simulink model "HouseHolderTransformTest"  (R2023b)
settings: Solver=VariableStepAuto  StartTime=0.0  StopTime=1  FixedStep=0.0038461538461538464  RelTol=1e-3
values from neighbouring files (symbols this model uses):
  A = [0.588528123101 -3.46944695195e-18 -8.67361737988e-19 0 0 6.93889390391e-18 6.93889390391e-18 6.93889390391e-18 1.38777878078e-17 0 0 6.93889390391e-18 ... (1040 elements, 260x4)]    [InitData.mat]
undefined symbols (not defined in the file or in its folder): FrameLength, NumOfAntennas
libraries: hdlsllib x5, dspstat3 x5
(part 1 of 2)
settings Model: Creator=Koche  LastModifiedBy=Koche
settings DebuggingCC: UnderSpecifiedDimensionMsg=error

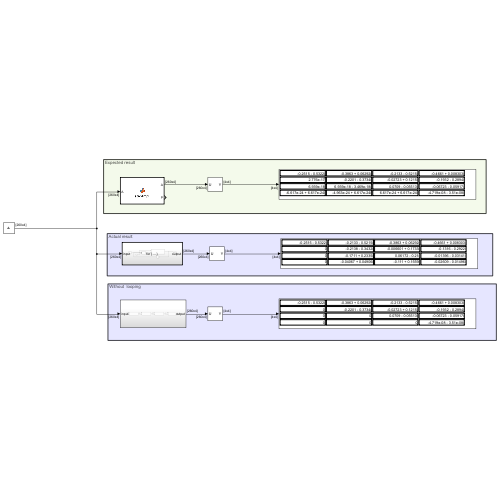
[thumbnail: Simulink's stored preview of the top-level diagram]
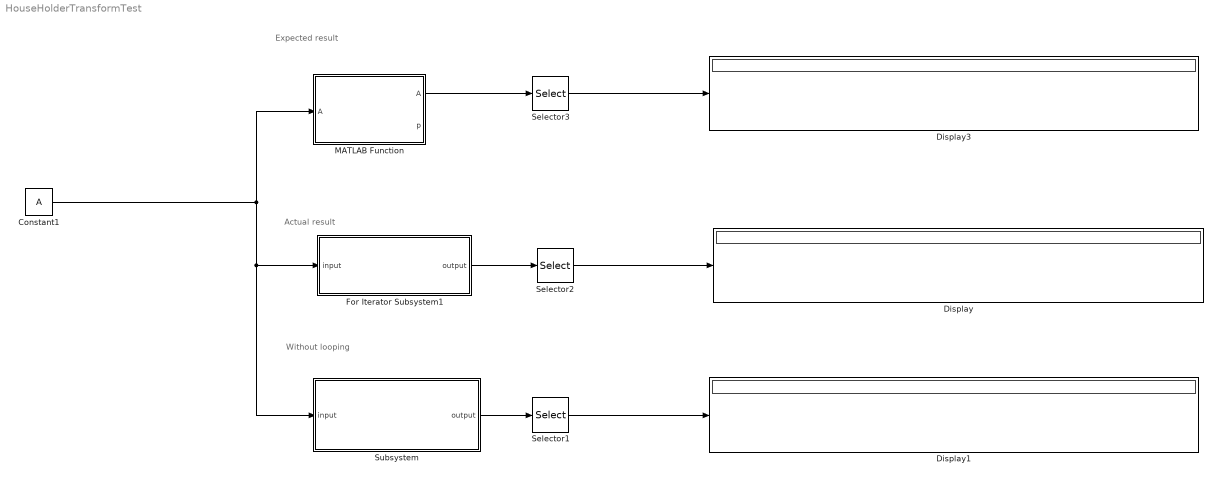
== system HouseHolderTransformTest ==
  note: Without looping
  note: Expected result
  note: Actual result
  Constant1 : Constant  Value=A  SampleTime=1/FrameLength
  Display : Display
  Display1 : Display
  Display3 : Display
  For Iterator Subsystem1 : Subsystem  TreatAsAtomicUnit=on
  MATLAB Function : MATLAB Function  TreatAsAtomicUnit=on
  Selector1 : Selector  NumberOfDimensions=2  InputPortWidth=3  IndexOptions=Index vector (dialog),Index vector (dialog)  Indices=[1 2 3 4],[1 2 3 4]  OutputSizes=1,1
  Selector2 : Selector  NumberOfDimensions=2  InputPortWidth=3  IndexOptions=Index vector (dialog),Index vector (dialog)  Indices=[1 2 3 4],[1 2 3 4]  OutputSizes=1,1
  Selector3 : Selector  NumberOfDimensions=2  InputPortWidth=3  IndexOptions=Index vector (dialog),Index vector (dialog)  Indices=[1 2 3 4],[1 2 3 4]  OutputSizes=1,1
  Subsystem : Subsystem
  wires:
  Constant1/1 -> Subsystem/1(input), For Iterator Subsystem1/1(input), MATLAB Function/1("A ")
  For Iterator Subsystem1/1(output) -> Selector2/1
  Selector2/1 -> Display/1
  Selector3/1 -> Display3/1
  MATLAB Function/1(A) -> Selector3/1
  Subsystem/1(output) -> Selector1/1
  Selector1/1 -> Display1/1

== system HouseHolderTransformTest/For Iterator Subsystem1 ==
  input : Inport
  For Iterator : ForIterator  IterationLimit=NumOfAntennas
  Memory1 : Memory  InheritSampleTime=on
  Subsystem3 : Subsystem
  Switch1 : Switch  Criteria=u2 > Threshold  Threshold=1  SaturateOnIntegerOverflow=off  InputSameDT=off
  output : Outport
  wires:
  input/1 -> Switch1/3
  Memory1/1 -> Switch1/1
  Switch1/1 -> Subsystem3/2(input)
  For Iterator/1 -> Subsystem3/1(n), Switch1/2
  Subsystem3/1(output) -> Memory1/1, output/1

== system HouseHolderTransformTest/Subsystem ==
  input : Inport
  Constant : Constant  OutDataTypeStr=int32
  Constant1 : Constant  Value=2  OutDataTypeStr=int32
  Constant2 : Constant  Value=3  OutDataTypeStr=int32
  Constant3 : Constant  Value=4  OutDataTypeStr=int32
  Subsystem1 : Subsystem
  Subsystem2 : Subsystem
  Subsystem3 : Subsystem
  Subsystem4 : Subsystem
  output : Outport
  wires:
  Constant/1 -> Subsystem3/1(n)
  Subsystem3/1(output) -> Subsystem1/2(input)
  Constant2/1 -> Subsystem2/1(n)
  Subsystem4/1(output) -> output/1
  Subsystem2/1(output) -> Subsystem4/2(input)
  Subsystem1/1(output) -> Subsystem2/2(input)
  input/1 -> Subsystem3/2(input)
  Constant3/1 -> Subsystem4/1(n)
  Constant1/1 -> Subsystem1/1(n)

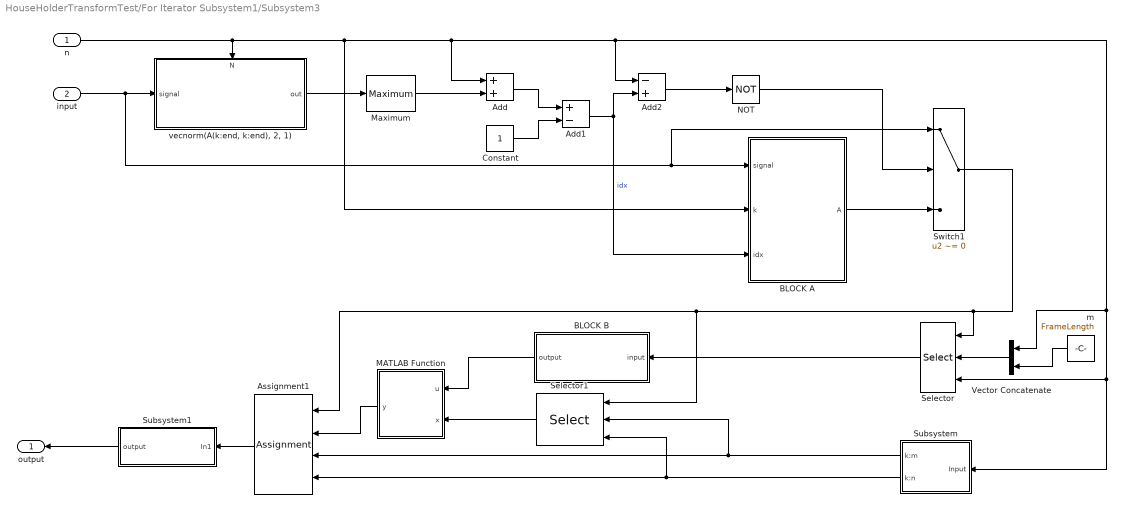
== system HouseHolderTransformTest/For Iterator Subsystem1/Subsystem3 ==
  n : Inport
  input : Inport  Port=2
  Add : Sum
  Add1 : Sum  Inputs=+-
  Add2 : Sum  Inputs=-+
  Assignment1 : Assignment  NumberOfDimensions=2  IndexOptions=Index vector (port),Index vector (port)  Indices=1,1  OutputSizes=1,1
  BLOCK A : Subsystem  TreatAsAtomicUnit=on
  BLOCK B : Subsystem
  Constant : Constant  SampleTime=-1
  MATLAB Function : MATLAB Function  TreatAsAtomicUnit=on
  Maximum : dspstat3/Maximum  operation=maximum  fcn=Index  indexBase=One  operateOver=Each column  Dimension=1  InputProcessing=Columns as channels (frame based)  reset=None  roiEnable=off  roiType=Rectangles  roiPortion=Entire ROI  roiOutput=Individual statistics for each ROI  roiFlag=off  roundingMode=Floor  overflowMode=off  accumDataTypeStr=Inherit: Same as product output  accumLastDataTypeStr=Inherit: Same as product output
      settings: LibrarySourceBlock=dsphdlsupportstat/Maximum
  NOT : Logic  Operator=NOT  IconShape=distinctive  AllPortsSameDT=off  OutDataTypeStr=boolean
  Selector : Selector  NumberOfDimensions=2  InputPortWidth=3  IndexOptions=Starting and ending indices (port),Index vector (port)  Indices=[1 3],1  OutputSizes=1,1
  Selector1 : Selector  NumberOfDimensions=2  InputPortWidth=3  IndexOptions=Index vector (port),Index vector (port)  Indices=[1 3],1  OutputSizes=1,1
  Subsystem : Subsystem
  Subsystem1 : Subsystem
  Switch1 : Switch  Criteria=u2 ~= 0  SaturateOnIntegerOverflow=off  InputSameDT=off
  Vector Concatenate : Concatenate
  m : Constant  Value=FrameLength  OutDataTypeStr=int32
  "vecnorm(A(k:end, k:end), 2, 1)" : Subsystem
      settings: PortSchema="{\"entries\":[{\"content\":{\"sides\":[{\"content\":{\"connectorIds\":[\"In1\"]},\"type\":\"ConnectorPlacement.EquallySpacedRectSide\",\"uuid\":\"ddbbb4e8-2c6c-4e6c-8e2e-3b3671634aad\"},{\"content\":{\"connectorIds\":[\"Out1\"],\"side\":\"RIGHT\"},\"type\":\"ConnectorPlacement.EquallySpacedRectSide\",\"uuid\":\"1781eb83-3214-4f0b-a111-2b3a2e27c9fb\"},{\"content\":{\"connectorIds\":[\"In2\"],\"side\":\"TOP\"},\"type\":\"ConnectorPlacement.EquallySpacedRectSide\",\"uuid\":\"ba31d641-ff62-4171-b945-e5cde8a84090\"}]},\"type\":\"ConnectorPlacement.EquallySpacedConnector\",\"uuid\":\"97f7897c-1f2b-447f-863d-894b57bebce4\"}],\"packageUris\":[\"http://schema.mathworks.com/mf0/Connector/R2020b\"],\"version\":\"1.0\"}"
  output : Outport
  wires:
  Add/1 -> Add1/1
  input/1 -> "vecnorm(A(k:end, k:end), 2, 1)"/1(signal), BLOCK A/1(signal), Switch1/1
  Maximum/1 -> Add/2
  Add1/1 -> Add2/2, BLOCK A/3(idx)  "idx"
  "vecnorm(A(k:end, k:end), 2, 1)"/1(out) -> Maximum/1
  Add2/1 -> NOT/1
  Constant/1 -> Add1/2
  NOT/1 -> Switch1/2
  BLOCK A/1(A) -> Switch1/3
  MATLAB Function/1(y) -> Assignment1/2
  Subsystem/2(k:n) -> Selector1/3, Assignment1/4
  Subsystem/1(k:m) -> Selector1/2, Assignment1/3
  n/1 -> "vecnorm(A(k:end, k:end), 2, 1)"/2(N), BLOCK A/2(k), Add/1, Add2/1, Subsystem/1(Input), Selector/3, Vector Concatenate/1
  Vector Concatenate/1 -> Selector/2
  Selector1/1 -> MATLAB Function/2(x)
  Switch1/1 -> Selector1/1, Assignment1/1, Selector/1
  BLOCK B/1(output) -> MATLAB Function/1(u)
  m/1 -> Vector Concatenate/2
  Selector/1 -> BLOCK B/1(input)
  Assignment1/1 -> Subsystem1/1(In1)
  Subsystem1/1(output) -> output/1

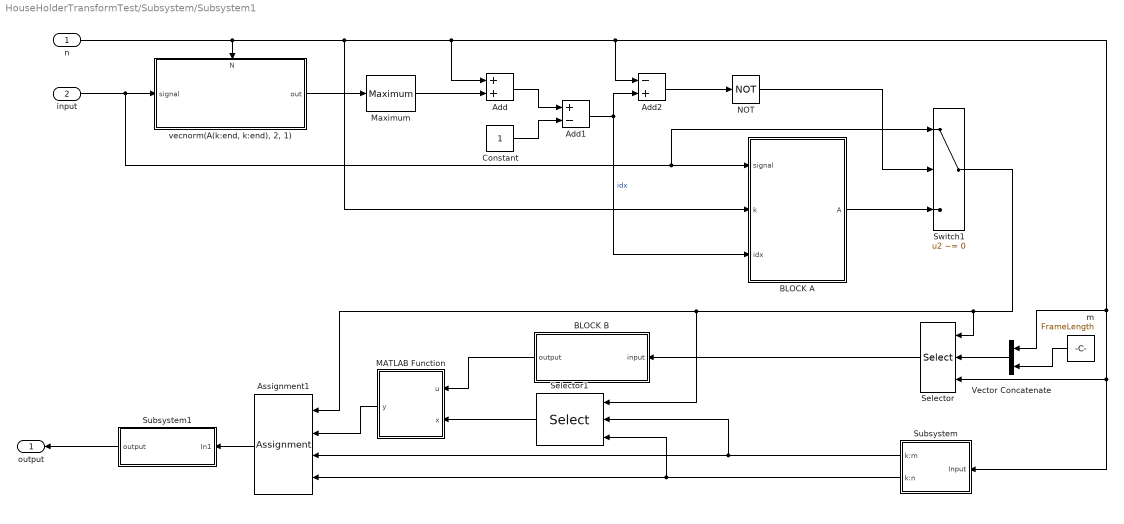
== system HouseHolderTransformTest/Subsystem/Subsystem1 ==
  n : Inport
  input : Inport  Port=2
  Add : Sum
  Add1 : Sum  Inputs=+-
  Add2 : Sum  Inputs=-+
  Assignment1 : Assignment  NumberOfDimensions=2  IndexOptions=Index vector (port),Index vector (port)  Indices=1,1  OutputSizes=1,1
  BLOCK A : Subsystem  TreatAsAtomicUnit=on
  BLOCK B : Subsystem
  Constant : Constant  SampleTime=-1
  MATLAB Function : MATLAB Function  TreatAsAtomicUnit=on
  Maximum : dspstat3/Maximum  operation=maximum  fcn=Index  indexBase=One  operateOver=Each column  Dimension=1  InputProcessing=Columns as channels (frame based)  reset=None  roiEnable=off  roiType=Rectangles  roiPortion=Entire ROI  roiOutput=Individual statistics for each ROI  roiFlag=off  roundingMode=Floor  overflowMode=off  accumDataTypeStr=Inherit: Same as product output  accumLastDataTypeStr=Inherit: Same as product output
      settings: LibrarySourceBlock=dsphdlsupportstat/Maximum
  NOT : Logic  Operator=NOT  IconShape=distinctive  AllPortsSameDT=off  OutDataTypeStr=boolean
  Selector : Selector  NumberOfDimensions=2  InputPortWidth=3  IndexOptions=Starting and ending indices (port),Index vector (port)  Indices=[1 3],1  OutputSizes=1,1
  Selector1 : Selector  NumberOfDimensions=2  InputPortWidth=3  IndexOptions=Index vector (port),Index vector (port)  Indices=[1 3],1  OutputSizes=1,1
  Subsystem : Subsystem
  Subsystem1 : Subsystem
  Switch1 : Switch  Criteria=u2 ~= 0  SaturateOnIntegerOverflow=off  InputSameDT=off
  Vector Concatenate : Concatenate
  m : Constant  Value=FrameLength  OutDataTypeStr=int32
  "vecnorm(A(k:end, k:end), 2, 1)" : Subsystem
      settings: PortSchema="{\"entries\":[{\"content\":{\"sides\":[{\"content\":{\"connectorIds\":[\"In1\"]},\"type\":\"ConnectorPlacement.EquallySpacedRectSide\",\"uuid\":\"ddbbb4e8-2c6c-4e6c-8e2e-3b3671634aad\"},{\"content\":{\"connectorIds\":[\"Out1\"],\"side\":\"RIGHT\"},\"type\":\"ConnectorPlacement.EquallySpacedRectSide\",\"uuid\":\"1781eb83-3214-4f0b-a111-2b3a2e27c9fb\"},{\"content\":{\"connectorIds\":[\"In2\"],\"side\":\"TOP\"},\"type\":\"ConnectorPlacement.EquallySpacedRectSide\",\"uuid\":\"ba31d641-ff62-4171-b945-e5cde8a84090\"}]},\"type\":\"ConnectorPlacement.EquallySpacedConnector\",\"uuid\":\"97f7897c-1f2b-447f-863d-894b57bebce4\"}],\"packageUris\":[\"http://schema.mathworks.com/mf0/Connector/R2020b\"],\"version\":\"1.0\"}"
  output : Outport
  wires:
  Subsystem1/1(output) -> output/1
  Assignment1/1 -> Subsystem1/1(In1)
  Selector/1 -> BLOCK B/1(input)
  m/1 -> Vector Concatenate/2
  BLOCK B/1(output) -> MATLAB Function/1(u)
  Switch1/1 -> Selector/1, Assignment1/1, Selector1/1
  Selector1/1 -> MATLAB Function/2(x)
  Vector Concatenate/1 -> Selector/2
  n/1 -> Vector Concatenate/1, Selector/3, Subsystem/1(Input), Add2/1, Add/1, BLOCK A/2(k), "vecnorm(A(k:end, k:end), 2, 1)"/2(N)
  Subsystem/1(k:m) -> Assignment1/3, Selector1/2
  Subsystem/2(k:n) -> Assignment1/4, Selector1/3
  MATLAB Function/1(y) -> Assignment1/2
  BLOCK A/1(A) -> Switch1/3
  NOT/1 -> Switch1/2
  Constant/1 -> Add1/2
  Add2/1 -> NOT/1
  "vecnorm(A(k:end, k:end), 2, 1)"/1(out) -> Maximum/1
  Add1/1 -> BLOCK A/3(idx), Add2/2  "idx"
  Maximum/1 -> Add/2
  input/1 -> Switch1/1, BLOCK A/1(signal), "vecnorm(A(k:end, k:end), 2, 1)"/1(signal)
  Add/1 -> Add1/1

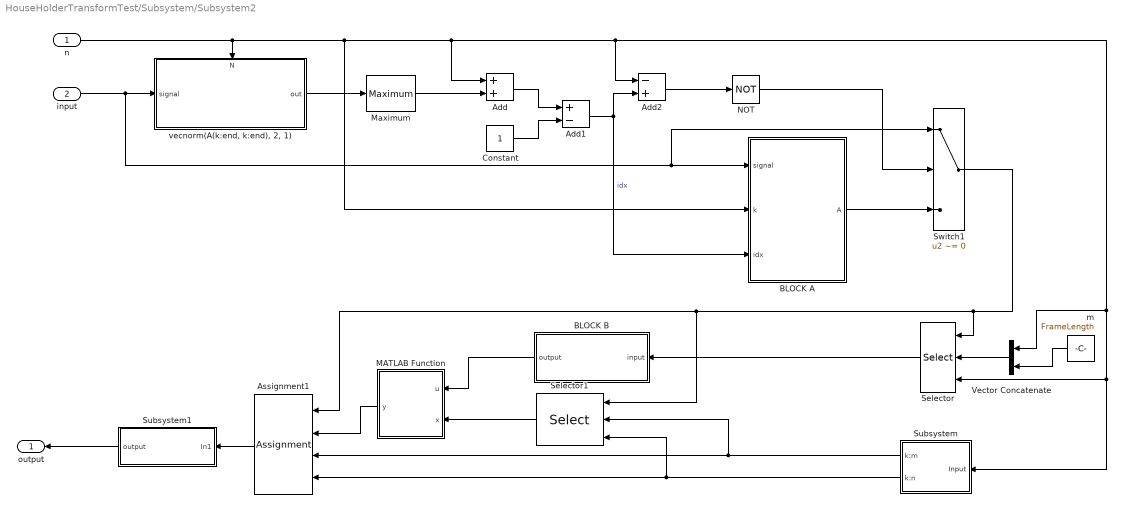
== system HouseHolderTransformTest/Subsystem/Subsystem2 ==
  n : Inport
  input : Inport  Port=2
  Add : Sum
  Add1 : Sum  Inputs=+-
  Add2 : Sum  Inputs=-+
  Assignment1 : Assignment  NumberOfDimensions=2  IndexOptions=Index vector (port),Index vector (port)  Indices=1,1  OutputSizes=1,1
  BLOCK A : Subsystem  TreatAsAtomicUnit=on
  BLOCK B : Subsystem
  Constant : Constant  SampleTime=-1
  MATLAB Function : MATLAB Function  TreatAsAtomicUnit=on
  Maximum : dspstat3/Maximum  operation=maximum  fcn=Index  indexBase=One  operateOver=Each column  Dimension=1  InputProcessing=Columns as channels (frame based)  reset=None  roiEnable=off  roiType=Rectangles  roiPortion=Entire ROI  roiOutput=Individual statistics for each ROI  roiFlag=off  roundingMode=Floor  overflowMode=off  accumDataTypeStr=Inherit: Same as product output  accumLastDataTypeStr=Inherit: Same as product output
      settings: LibrarySourceBlock=dsphdlsupportstat/Maximum
  NOT : Logic  Operator=NOT  IconShape=distinctive  AllPortsSameDT=off  OutDataTypeStr=boolean
  Selector : Selector  NumberOfDimensions=2  InputPortWidth=3  IndexOptions=Starting and ending indices (port),Index vector (port)  Indices=[1 3],1  OutputSizes=1,1
  Selector1 : Selector  NumberOfDimensions=2  InputPortWidth=3  IndexOptions=Index vector (port),Index vector (port)  Indices=[1 3],1  OutputSizes=1,1
  Subsystem : Subsystem
  Subsystem1 : Subsystem
  Switch1 : Switch  Criteria=u2 ~= 0  SaturateOnIntegerOverflow=off  InputSameDT=off
  Vector Concatenate : Concatenate
  m : Constant  Value=FrameLength  OutDataTypeStr=int32
  "vecnorm(A(k:end, k:end), 2, 1)" : Subsystem
      settings: PortSchema="{\"entries\":[{\"content\":{\"sides\":[{\"content\":{\"connectorIds\":[\"In1\"]},\"type\":\"ConnectorPlacement.EquallySpacedRectSide\",\"uuid\":\"ddbbb4e8-2c6c-4e6c-8e2e-3b3671634aad\"},{\"content\":{\"connectorIds\":[\"Out1\"],\"side\":\"RIGHT\"},\"type\":\"ConnectorPlacement.EquallySpacedRectSide\",\"uuid\":\"1781eb83-3214-4f0b-a111-2b3a2e27c9fb\"},{\"content\":{\"connectorIds\":[\"In2\"],\"side\":\"TOP\"},\"type\":\"ConnectorPlacement.EquallySpacedRectSide\",\"uuid\":\"ba31d641-ff62-4171-b945-e5cde8a84090\"}]},\"type\":\"ConnectorPlacement.EquallySpacedConnector\",\"uuid\":\"97f7897c-1f2b-447f-863d-894b57bebce4\"}],\"packageUris\":[\"http://schema.mathworks.com/mf0/Connector/R2020b\"],\"version\":\"1.0\"}"
  output : Outport
  wires:
  Add/1 -> Add1/1
  input/1 -> "vecnorm(A(k:end, k:end), 2, 1)"/1(signal), BLOCK A/1(signal), Switch1/1
  Maximum/1 -> Add/2
  Add1/1 -> Add2/2, BLOCK A/3(idx)  "idx"
  "vecnorm(A(k:end, k:end), 2, 1)"/1(out) -> Maximum/1
  Add2/1 -> NOT/1
  Constant/1 -> Add1/2
  NOT/1 -> Switch1/2
  BLOCK A/1(A) -> Switch1/3
  MATLAB Function/1(y) -> Assignment1/2
  Subsystem/2(k:n) -> Selector1/3, Assignment1/4
  Subsystem/1(k:m) -> Selector1/2, Assignment1/3
  n/1 -> "vecnorm(A(k:end, k:end), 2, 1)"/2(N), BLOCK A/2(k), Add/1, Add2/1, Subsystem/1(Input), Selector/3, Vector Concatenate/1
  Vector Concatenate/1 -> Selector/2
  Selector1/1 -> MATLAB Function/2(x)
  Switch1/1 -> Selector1/1, Assignment1/1, Selector/1
  BLOCK B/1(output) -> MATLAB Function/1(u)
  m/1 -> Vector Concatenate/2
  Selector/1 -> BLOCK B/1(input)
  Assignment1/1 -> Subsystem1/1(In1)
  Subsystem1/1(output) -> output/1

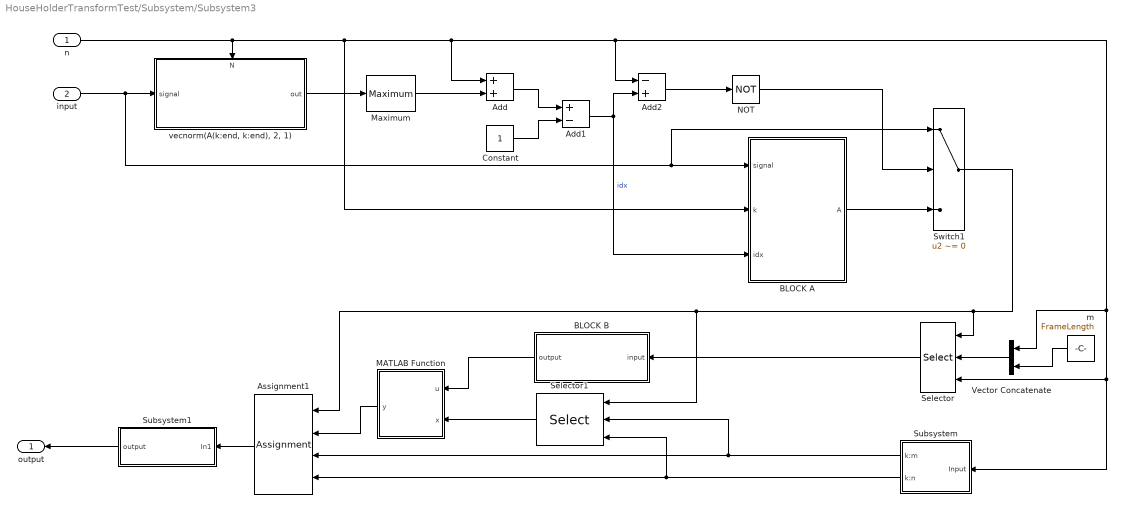
== system HouseHolderTransformTest/Subsystem/Subsystem3 ==
  n : Inport
  input : Inport  Port=2
  Add : Sum
  Add1 : Sum  Inputs=+-
  Add2 : Sum  Inputs=-+
  Assignment1 : Assignment  NumberOfDimensions=2  IndexOptions=Index vector (port),Index vector (port)  Indices=1,1  OutputSizes=1,1
  BLOCK A : Subsystem  TreatAsAtomicUnit=on
  BLOCK B : Subsystem
  Constant : Constant  SampleTime=-1
  MATLAB Function : MATLAB Function  TreatAsAtomicUnit=on
  Maximum : dspstat3/Maximum  operation=maximum  fcn=Index  indexBase=One  operateOver=Each column  Dimension=1  InputProcessing=Columns as channels (frame based)  reset=None  roiEnable=off  roiType=Rectangles  roiPortion=Entire ROI  roiOutput=Individual statistics for each ROI  roiFlag=off  roundingMode=Floor  overflowMode=off  accumDataTypeStr=Inherit: Same as product output  accumLastDataTypeStr=Inherit: Same as product output
      settings: LibrarySourceBlock=dsphdlsupportstat/Maximum
  NOT : Logic  Operator=NOT  IconShape=distinctive  AllPortsSameDT=off  OutDataTypeStr=boolean
  Selector : Selector  NumberOfDimensions=2  InputPortWidth=3  IndexOptions=Starting and ending indices (port),Index vector (port)  Indices=[1 3],1  OutputSizes=1,1
  Selector1 : Selector  NumberOfDimensions=2  InputPortWidth=3  IndexOptions=Index vector (port),Index vector (port)  Indices=[1 3],1  OutputSizes=1,1
  Subsystem : Subsystem
  Subsystem1 : Subsystem
  Switch1 : Switch  Criteria=u2 ~= 0  SaturateOnIntegerOverflow=off  InputSameDT=off
  Vector Concatenate : Concatenate
  m : Constant  Value=FrameLength  OutDataTypeStr=int32
  "vecnorm(A(k:end, k:end), 2, 1)" : Subsystem
      settings: PortSchema="{\"entries\":[{\"content\":{\"sides\":[{\"content\":{\"connectorIds\":[\"In1\"]},\"type\":\"ConnectorPlacement.EquallySpacedRectSide\",\"uuid\":\"ddbbb4e8-2c6c-4e6c-8e2e-3b3671634aad\"},{\"content\":{\"connectorIds\":[\"Out1\"],\"side\":\"RIGHT\"},\"type\":\"ConnectorPlacement.EquallySpacedRectSide\",\"uuid\":\"1781eb83-3214-4f0b-a111-2b3a2e27c9fb\"},{\"content\":{\"connectorIds\":[\"In2\"],\"side\":\"TOP\"},\"type\":\"ConnectorPlacement.EquallySpacedRectSide\",\"uuid\":\"ba31d641-ff62-4171-b945-e5cde8a84090\"}]},\"type\":\"ConnectorPlacement.EquallySpacedConnector\",\"uuid\":\"97f7897c-1f2b-447f-863d-894b57bebce4\"}],\"packageUris\":[\"http://schema.mathworks.com/mf0/Connector/R2020b\"],\"version\":\"1.0\"}"
  output : Outport
  wires:
  Add/1 -> Add1/1
  input/1 -> "vecnorm(A(k:end, k:end), 2, 1)"/1(signal), BLOCK A/1(signal), Switch1/1
  Maximum/1 -> Add/2
  Add1/1 -> Add2/2, BLOCK A/3(idx)  "idx"
  "vecnorm(A(k:end, k:end), 2, 1)"/1(out) -> Maximum/1
  Add2/1 -> NOT/1
  Constant/1 -> Add1/2
  NOT/1 -> Switch1/2
  BLOCK A/1(A) -> Switch1/3
  MATLAB Function/1(y) -> Assignment1/2
  Subsystem/2(k:n) -> Selector1/3, Assignment1/4
  Subsystem/1(k:m) -> Selector1/2, Assignment1/3
  n/1 -> "vecnorm(A(k:end, k:end), 2, 1)"/2(N), BLOCK A/2(k), Add/1, Add2/1, Subsystem/1(Input), Selector/3, Vector Concatenate/1
  Vector Concatenate/1 -> Selector/2
  Selector1/1 -> MATLAB Function/2(x)
  Switch1/1 -> Selector1/1, Assignment1/1, Selector/1
  BLOCK B/1(output) -> MATLAB Function/1(u)
  m/1 -> Vector Concatenate/2
  Selector/1 -> BLOCK B/1(input)
  Assignment1/1 -> Subsystem1/1(In1)
  Subsystem1/1(output) -> output/1

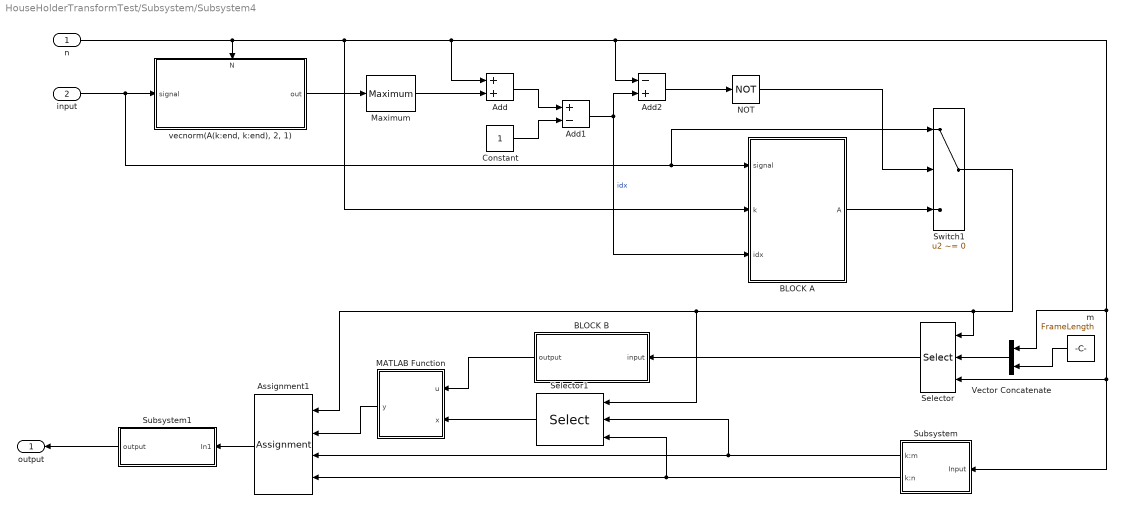
== system HouseHolderTransformTest/Subsystem/Subsystem4 ==
  n : Inport
  input : Inport  Port=2
  Add : Sum
  Add1 : Sum  Inputs=+-
  Add2 : Sum  Inputs=-+
  Assignment1 : Assignment  NumberOfDimensions=2  IndexOptions=Index vector (port),Index vector (port)  Indices=1,1  OutputSizes=1,1
  BLOCK A : Subsystem  TreatAsAtomicUnit=on
  BLOCK B : Subsystem
  Constant : Constant  SampleTime=-1
  MATLAB Function : MATLAB Function  TreatAsAtomicUnit=on
  Maximum : dspstat3/Maximum  operation=maximum  fcn=Index  indexBase=One  operateOver=Each column  Dimension=1  InputProcessing=Columns as channels (frame based)  reset=None  roiEnable=off  roiType=Rectangles  roiPortion=Entire ROI  roiOutput=Individual statistics for each ROI  roiFlag=off  roundingMode=Floor  overflowMode=off  accumDataTypeStr=Inherit: Same as product output  accumLastDataTypeStr=Inherit: Same as product output
      settings: LibrarySourceBlock=dsphdlsupportstat/Maximum
  NOT : Logic  Operator=NOT  IconShape=distinctive  AllPortsSameDT=off  OutDataTypeStr=boolean
  Selector : Selector  NumberOfDimensions=2  InputPortWidth=3  IndexOptions=Starting and ending indices (port),Index vector (port)  Indices=[1 3],1  OutputSizes=1,1
  Selector1 : Selector  NumberOfDimensions=2  InputPortWidth=3  IndexOptions=Index vector (port),Index vector (port)  Indices=[1 3],1  OutputSizes=1,1
  Subsystem : Subsystem
  Subsystem1 : Subsystem
  Switch1 : Switch  Criteria=u2 ~= 0  SaturateOnIntegerOverflow=off  InputSameDT=off
  Vector Concatenate : Concatenate
  m : Constant  Value=FrameLength  OutDataTypeStr=int32
  "vecnorm(A(k:end, k:end), 2, 1)" : Subsystem
      settings: PortSchema="{\"entries\":[{\"content\":{\"sides\":[{\"content\":{\"connectorIds\":[\"In1\"]},\"type\":\"ConnectorPlacement.EquallySpacedRectSide\",\"uuid\":\"ddbbb4e8-2c6c-4e6c-8e2e-3b3671634aad\"},{\"content\":{\"connectorIds\":[\"Out1\"],\"side\":\"RIGHT\"},\"type\":\"ConnectorPlacement.EquallySpacedRectSide\",\"uuid\":\"1781eb83-3214-4f0b-a111-2b3a2e27c9fb\"},{\"content\":{\"connectorIds\":[\"In2\"],\"side\":\"TOP\"},\"type\":\"ConnectorPlacement.EquallySpacedRectSide\",\"uuid\":\"ba31d641-ff62-4171-b945-e5cde8a84090\"}]},\"type\":\"ConnectorPlacement.EquallySpacedConnector\",\"uuid\":\"97f7897c-1f2b-447f-863d-894b57bebce4\"}],\"packageUris\":[\"http://schema.mathworks.com/mf0/Connector/R2020b\"],\"version\":\"1.0\"}"
  output : Outport
  wires:
  Subsystem1/1(output) -> output/1
  Assignment1/1 -> Subsystem1/1(In1)
  Selector/1 -> BLOCK B/1(input)
  m/1 -> Vector Concatenate/2
  BLOCK B/1(output) -> MATLAB Function/1(u)
  Switch1/1 -> Selector/1, Assignment1/1, Selector1/1
  Selector1/1 -> MATLAB Function/2(x)
  Vector Concatenate/1 -> Selector/2
  n/1 -> Vector Concatenate/1, Selector/3, Subsystem/1(Input), Add2/1, Add/1, BLOCK A/2(k), "vecnorm(A(k:end, k:end), 2, 1)"/2(N)
  Subsystem/1(k:m) -> Assignment1/3, Selector1/2
  Subsystem/2(k:n) -> Assignment1/4, Selector1/3
  MATLAB Function/1(y) -> Assignment1/2
  BLOCK A/1(A) -> Switch1/3
  NOT/1 -> Switch1/2
  Constant/1 -> Add1/2
  Add2/1 -> NOT/1
  "vecnorm(A(k:end, k:end), 2, 1)"/1(out) -> Maximum/1
  Add1/1 -> BLOCK A/3(idx), Add2/2  "idx"
  Maximum/1 -> Add/2
  input/1 -> Switch1/1, BLOCK A/1(signal), "vecnorm(A(k:end, k:end), 2, 1)"/1(signal)
  Add/1 -> Add1/1

== system HouseHolderTransformTest/For Iterator Subsystem1/Subsystem3/BLOCK A ==
  signal : Inport
  k : Inport  Port=2
  idx : Inport  Port=3
  MATLAB Function : MATLAB Function  TreatAsAtomicUnit=on
  A : Outport
  wires:
  idx/1 -> MATLAB Function/2(idx)
  k/1 -> MATLAB Function/3(k)
  MATLAB Function/1(A) -> A/1
  signal/1 -> MATLAB Function/1("A ")

== system HouseHolderTransformTest/For Iterator Subsystem1/Subsystem3/BLOCK B ==
  input : Inport
  2nd Norm : Subsystem
  If Action Subsystem : Subsystem  TreatAsAtomicUnit=on
  If Action Subsystem1 : Subsystem  TreatAsAtomicUnit=on
  Switch : Switch  Criteria=u2 ~= 0  AllowDiffInputSizes=on  SaturateOnIntegerOverflow=off  InputSameDT=off
  output : Outport
  wires:
  input/1 -> If Action Subsystem1/1(x), If Action Subsystem/2(x), 2nd Norm/1(input)
  If Action Subsystem1/1(u) -> Switch/3
  Switch/1 -> output/1
  If Action Subsystem/1(u) -> Switch/1
  2nd Norm/1(output) -> Switch/2, If Action Subsystem/1(norm)  "normX"

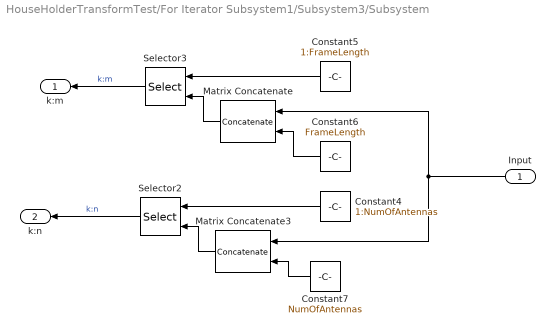
== system HouseHolderTransformTest/For Iterator Subsystem1/Subsystem3/Subsystem ==
  Input : Inport
  Constant4 : Constant  Value=1:NumOfAntennas  OutDataTypeStr=int32  SampleTime=-1
  Constant5 : Constant  Value=1:FrameLength  OutDataTypeStr=int32  SampleTime=-1
  Constant6 : Constant  Value=FrameLength  OutDataTypeStr=int32
  Constant7 : Constant  Value=NumOfAntennas  OutDataTypeStr=int32
  Matrix Concatenate : Concatenate  Mode=Multidimensional array
  Matrix Concatenate3 : Concatenate  Mode=Multidimensional array
  Selector2 : Selector  IndexOptions=Starting and ending indices (port)  Indices=[1 3]  OutputSizes=1
  Selector3 : Selector  IndexOptions=Starting and ending indices (port)  Indices=[1 3]  OutputSizes=1
  k:m : Outport
  k:n : Outport  Port=2
  wires:
  Input/1 -> Matrix Concatenate3/1, Matrix Concatenate/1
  Selector3/1 -> k:m/1  "k:m"
  Selector2/1 -> k:n/1  "k:n"
  Constant6/1 -> Matrix Concatenate/2
  Matrix Concatenate/1 -> Selector3/2
  Constant7/1 -> Matrix Concatenate3/2
  Constant4/1 -> Selector2/1
  Matrix Concatenate3/1 -> Selector2/2
  Constant5/1 -> Selector3/1

== system HouseHolderTransformTest/For Iterator Subsystem1/Subsystem3/Subsystem1 ==
  In1 : Inport
  Abs : Abs  SaturateOnIntegerOverflow=off
  Abs1 : Abs  SaturateOnIntegerOverflow=off
  Complex to Real-Imag : ComplexToRealImag
  Constant : Constant  Value=0
  Constant1 : Constant  Value=0
  Real-Imag to Complex : RealImagToComplex
  Switch : Switch  Criteria=u2 > Threshold  Threshold=1e-10  SaturateOnIntegerOverflow=off  InputSameDT=off
  Switch1 : Switch  Criteria=u2 > Threshold  Threshold=1e-10  SaturateOnIntegerOverflow=off  InputSameDT=off
  output : Outport
  wires:
  In1/1 -> Complex to Real-Imag/1
  Complex to Real-Imag/1 -> Abs/1, Switch/1
  Constant/1 -> Switch/3
  Constant1/1 -> Switch1/3
  Complex to Real-Imag/2 -> Abs1/1, Switch1/1
  Switch/1 -> Real-Imag to Complex/1
  Switch1/1 -> Real-Imag to Complex/2
  Real-Imag to Complex/1 -> output/1
  Abs/1 -> Switch/2
  Abs1/1 -> Switch1/2

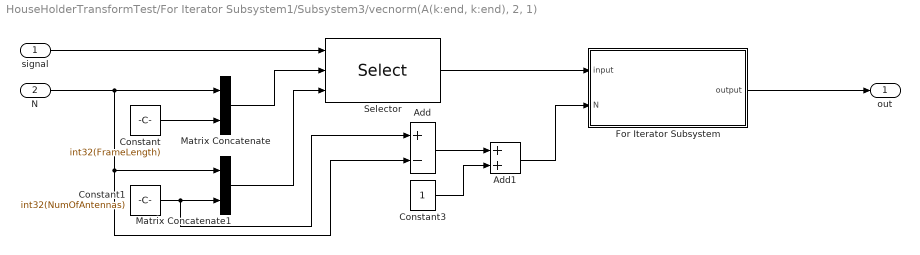
== system HouseHolderTransformTest/For Iterator Subsystem1/Subsystem3/vecnorm(A(k:end, k:end), 2, 1) ==
  signal : Inport
  N : Inport  Port=2
  Add : Sum  Inputs=+-
  Add1 : Sum
  Constant : Constant  Value=int32(FrameLength)  SampleTime=-1
  Constant1 : Constant  Value=int32(NumOfAntennas)  SampleTime=-1
  Constant3 : Constant
  For Iterator Subsystem : Subsystem  TreatAsAtomicUnit=on
  Matrix Concatenate : Concatenate
  Matrix Concatenate1 : Concatenate
  Selector : Selector  NumberOfDimensions=2  InputPortWidth=3  IndexOptions=Starting and ending indices (port),Starting and ending indices (port)  Indices=[1 3],1  OutputSizes=1,1
  out : Outport
  wires:
  Selector/1 -> For Iterator Subsystem/1(input)
  Add1/1 -> For Iterator Subsystem/2(N)
  For Iterator Subsystem/1(output) -> out/1
  Constant3/1 -> Add1/2
  Add/1 -> Add1/1
  N/1 -> Matrix Concatenate/1, Add/2, Matrix Concatenate1/1
  Constant1/1 -> Matrix Concatenate1/2, Add/1
  Matrix Concatenate1/1 -> Selector/3
  Constant/1 -> Matrix Concatenate/2
  Matrix Concatenate/1 -> Selector/2
  signal/1 -> Selector/1

== system HouseHolderTransformTest/Subsystem/Subsystem1/BLOCK A ==
  signal : Inport
  k : Inport  Port=2
  idx : Inport  Port=3
  MATLAB Function : MATLAB Function  TreatAsAtomicUnit=on
  A : Outport
  wires:
  signal/1 -> MATLAB Function/1("A ")
  MATLAB Function/1(A) -> A/1
  k/1 -> MATLAB Function/3(k)
  idx/1 -> MATLAB Function/2(idx)

== system HouseHolderTransformTest/Subsystem/Subsystem1/BLOCK B ==
  input : Inport
  2nd Norm : Subsystem
  If Action Subsystem : Subsystem  TreatAsAtomicUnit=on
  If Action Subsystem1 : Subsystem  TreatAsAtomicUnit=on
  Switch : Switch  Criteria=u2 ~= 0  AllowDiffInputSizes=on  SaturateOnIntegerOverflow=off  InputSameDT=off
  output : Outport
  wires:
  2nd Norm/1(output) -> If Action Subsystem/1(norm), Switch/2  "normX"
  If Action Subsystem/1(u) -> Switch/1
  Switch/1 -> output/1
  If Action Subsystem1/1(u) -> Switch/3
  input/1 -> 2nd Norm/1(input), If Action Subsystem/2(x), If Action Subsystem1/1(x)

== system HouseHolderTransformTest/Subsystem/Subsystem1/Subsystem ==
  Input : Inport
  Constant4 : Constant  Value=1:NumOfAntennas  OutDataTypeStr=int32  SampleTime=-1
  Constant5 : Constant  Value=1:FrameLength  OutDataTypeStr=int32  SampleTime=-1
  Constant6 : Constant  Value=FrameLength  OutDataTypeStr=int32
  Constant7 : Constant  Value=NumOfAntennas  OutDataTypeStr=int32
  Matrix Concatenate : Concatenate  Mode=Multidimensional array
  Matrix Concatenate3 : Concatenate  Mode=Multidimensional array
  Selector2 : Selector  IndexOptions=Starting and ending indices (port)  Indices=[1 3]  OutputSizes=1
  Selector3 : Selector  IndexOptions=Starting and ending indices (port)  Indices=[1 3]  OutputSizes=1
  k:m : Outport
  k:n : Outport  Port=2
  wires:
  Constant5/1 -> Selector3/1
  Matrix Concatenate3/1 -> Selector2/2
  Constant4/1 -> Selector2/1
  Constant7/1 -> Matrix Concatenate3/2
  Matrix Concatenate/1 -> Selector3/2
  Constant6/1 -> Matrix Concatenate/2
  Selector2/1 -> k:n/1  "k:n"
  Selector3/1 -> k:m/1  "k:m"
  Input/1 -> Matrix Concatenate/1, Matrix Concatenate3/1

== system HouseHolderTransformTest/Subsystem/Subsystem1/Subsystem1 ==
  In1 : Inport
  Abs : Abs  SaturateOnIntegerOverflow=off
  Abs1 : Abs  SaturateOnIntegerOverflow=off
  Complex to Real-Imag : ComplexToRealImag
  Constant : Constant  Value=0
  Constant1 : Constant  Value=0
  Real-Imag to Complex : RealImagToComplex
  Switch : Switch  Criteria=u2 > Threshold  Threshold=1e-10  SaturateOnIntegerOverflow=off  InputSameDT=off
  Switch1 : Switch  Criteria=u2 > Threshold  Threshold=1e-10  SaturateOnIntegerOverflow=off  InputSameDT=off
  output : Outport
  wires:
  Abs1/1 -> Switch1/2
  Abs/1 -> Switch/2
  Real-Imag to Complex/1 -> output/1
  Switch1/1 -> Real-Imag to Complex/2
  Switch/1 -> Real-Imag to Complex/1
  Complex to Real-Imag/2 -> Switch1/1, Abs1/1
  Constant1/1 -> Switch1/3
  Constant/1 -> Switch/3
  Complex to Real-Imag/1 -> Switch/1, Abs/1
  In1/1 -> Complex to Real-Imag/1

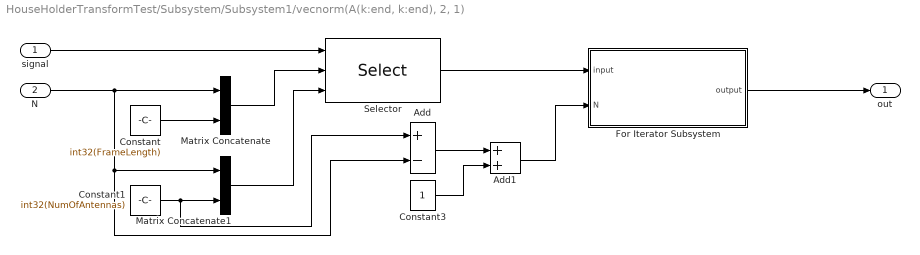
== system HouseHolderTransformTest/Subsystem/Subsystem1/vecnorm(A(k:end, k:end), 2, 1) ==
  signal : Inport
  N : Inport  Port=2
  Add : Sum  Inputs=+-
  Add1 : Sum
  Constant : Constant  Value=int32(FrameLength)  SampleTime=-1
  Constant1 : Constant  Value=int32(NumOfAntennas)  SampleTime=-1
  Constant3 : Constant
  For Iterator Subsystem : Subsystem  TreatAsAtomicUnit=on
  Matrix Concatenate : Concatenate
  Matrix Concatenate1 : Concatenate
  Selector : Selector  NumberOfDimensions=2  InputPortWidth=3  IndexOptions=Starting and ending indices (port),Starting and ending indices (port)  Indices=[1 3],1  OutputSizes=1,1
  out : Outport
  wires:
  signal/1 -> Selector/1
  Matrix Concatenate/1 -> Selector/2
  Constant/1 -> Matrix Concatenate/2
  Matrix Concatenate1/1 -> Selector/3
  Constant1/1 -> Add/1, Matrix Concatenate1/2
  N/1 -> Matrix Concatenate1/1, Add/2, Matrix Concatenate/1
  Add/1 -> Add1/1
  Constant3/1 -> Add1/2
  For Iterator Subsystem/1(output) -> out/1
  Add1/1 -> For Iterator Subsystem/2(N)
  Selector/1 -> For Iterator Subsystem/1(input)

== system HouseHolderTransformTest/Subsystem/Subsystem2/BLOCK A ==
  signal : Inport
  k : Inport  Port=2
  idx : Inport  Port=3
  MATLAB Function : MATLAB Function  TreatAsAtomicUnit=on
  A : Outport
  wires:
  idx/1 -> MATLAB Function/2(idx)
  k/1 -> MATLAB Function/3(k)
  MATLAB Function/1(A) -> A/1
  signal/1 -> MATLAB Function/1("A ")

== system HouseHolderTransformTest/Subsystem/Subsystem2/BLOCK B ==
  input : Inport
  2nd Norm : Subsystem
  If Action Subsystem : Subsystem  TreatAsAtomicUnit=on
  If Action Subsystem1 : Subsystem  TreatAsAtomicUnit=on
  Switch : Switch  Criteria=u2 ~= 0  AllowDiffInputSizes=on  SaturateOnIntegerOverflow=off  InputSameDT=off
  output : Outport
  wires:
  input/1 -> If Action Subsystem1/1(x), If Action Subsystem/2(x), 2nd Norm/1(input)
  If Action Subsystem1/1(u) -> Switch/3
  Switch/1 -> output/1
  If Action Subsystem/1(u) -> Switch/1
  2nd Norm/1(output) -> Switch/2, If Action Subsystem/1(norm)  "normX"

== system HouseHolderTransformTest/Subsystem/Subsystem2/Subsystem ==
  Input : Inport
  Constant4 : Constant  Value=1:NumOfAntennas  OutDataTypeStr=int32  SampleTime=-1
  Constant5 : Constant  Value=1:FrameLength  OutDataTypeStr=int32  SampleTime=-1
  Constant6 : Constant  Value=FrameLength  OutDataTypeStr=int32
  Constant7 : Constant  Value=NumOfAntennas  OutDataTypeStr=int32
  Matrix Concatenate : Concatenate  Mode=Multidimensional array
  Matrix Concatenate3 : Concatenate  Mode=Multidimensional array
  Selector2 : Selector  IndexOptions=Starting and ending indices (port)  Indices=[1 3]  OutputSizes=1
  Selector3 : Selector  IndexOptions=Starting and ending indices (port)  Indices=[1 3]  OutputSizes=1
  k:m : Outport
  k:n : Outport  Port=2
  wires:
  Input/1 -> Matrix Concatenate3/1, Matrix Concatenate/1
  Selector3/1 -> k:m/1  "k:m"
  Selector2/1 -> k:n/1  "k:n"
  Constant6/1 -> Matrix Concatenate/2
  Matrix Concatenate/1 -> Selector3/2
  Constant7/1 -> Matrix Concatenate3/2
  Constant4/1 -> Selector2/1
  Matrix Concatenate3/1 -> Selector2/2
  Constant5/1 -> Selector3/1

== system HouseHolderTransformTest/Subsystem/Subsystem2/Subsystem1 ==
  In1 : Inport
  Abs : Abs  SaturateOnIntegerOverflow=off
  Abs1 : Abs  SaturateOnIntegerOverflow=off
  Complex to Real-Imag : ComplexToRealImag
  Constant : Constant  Value=0
  Constant1 : Constant  Value=0
  Real-Imag to Complex : RealImagToComplex
  Switch : Switch  Criteria=u2 > Threshold  Threshold=1e-10  SaturateOnIntegerOverflow=off  InputSameDT=off
  Switch1 : Switch  Criteria=u2 > Threshold  Threshold=1e-10  SaturateOnIntegerOverflow=off  InputSameDT=off
  output : Outport
  wires:
  In1/1 -> Complex to Real-Imag/1
  Complex to Real-Imag/1 -> Abs/1, Switch/1
  Constant/1 -> Switch/3
  Constant1/1 -> Switch1/3
  Complex to Real-Imag/2 -> Abs1/1, Switch1/1
  Switch/1 -> Real-Imag to Complex/1
  Switch1/1 -> Real-Imag to Complex/2
  Real-Imag to Complex/1 -> output/1
  Abs/1 -> Switch/2
  Abs1/1 -> Switch1/2

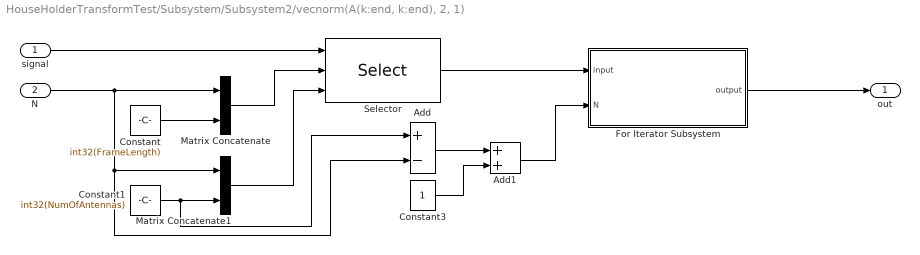
== system HouseHolderTransformTest/Subsystem/Subsystem2/vecnorm(A(k:end, k:end), 2, 1) ==
  signal : Inport
  N : Inport  Port=2
  Add : Sum  Inputs=+-
  Add1 : Sum
  Constant : Constant  Value=int32(FrameLength)  SampleTime=-1
  Constant1 : Constant  Value=int32(NumOfAntennas)  SampleTime=-1
  Constant3 : Constant
  For Iterator Subsystem : Subsystem  TreatAsAtomicUnit=on
  Matrix Concatenate : Concatenate
  Matrix Concatenate1 : Concatenate
  Selector : Selector  NumberOfDimensions=2  InputPortWidth=3  IndexOptions=Starting and ending indices (port),Starting and ending indices (port)  Indices=[1 3],1  OutputSizes=1,1
  out : Outport
  wires:
  Selector/1 -> For Iterator Subsystem/1(input)
  Add1/1 -> For Iterator Subsystem/2(N)
  For Iterator Subsystem/1(output) -> out/1
  Constant3/1 -> Add1/2
  Add/1 -> Add1/1
  N/1 -> Matrix Concatenate/1, Add/2, Matrix Concatenate1/1
  Constant1/1 -> Matrix Concatenate1/2, Add/1
  Matrix Concatenate1/1 -> Selector/3
  Constant/1 -> Matrix Concatenate/2
  Matrix Concatenate/1 -> Selector/2
  signal/1 -> Selector/1

== system HouseHolderTransformTest/Subsystem/Subsystem3/BLOCK A ==
  signal : Inport
  k : Inport  Port=2
  idx : Inport  Port=3
  MATLAB Function : MATLAB Function  TreatAsAtomicUnit=on
  A : Outport
  wires:
  idx/1 -> MATLAB Function/2(idx)
  k/1 -> MATLAB Function/3(k)
  MATLAB Function/1(A) -> A/1
  signal/1 -> MATLAB Function/1("A ")

== system HouseHolderTransformTest/Subsystem/Subsystem3/BLOCK B ==
  input : Inport
  2nd Norm : Subsystem
  If Action Subsystem : Subsystem  TreatAsAtomicUnit=on
  If Action Subsystem1 : Subsystem  TreatAsAtomicUnit=on
  Switch : Switch  Criteria=u2 ~= 0  AllowDiffInputSizes=on  SaturateOnIntegerOverflow=off  InputSameDT=off
  output : Outport
  wires:
  input/1 -> If Action Subsystem1/1(x), If Action Subsystem/2(x), 2nd Norm/1(input)
  If Action Subsystem1/1(u) -> Switch/3
  Switch/1 -> output/1
  If Action Subsystem/1(u) -> Switch/1
  2nd Norm/1(output) -> Switch/2, If Action Subsystem/1(norm)  "normX"

== system HouseHolderTransformTest/Subsystem/Subsystem3/Subsystem ==
  Input : Inport
  Constant4 : Constant  Value=1:NumOfAntennas  OutDataTypeStr=int32  SampleTime=-1
  Constant5 : Constant  Value=1:FrameLength  OutDataTypeStr=int32  SampleTime=-1
  Constant6 : Constant  Value=FrameLength  OutDataTypeStr=int32
  Constant7 : Constant  Value=NumOfAntennas  OutDataTypeStr=int32
  Matrix Concatenate : Concatenate  Mode=Multidimensional array
  Matrix Concatenate3 : Concatenate  Mode=Multidimensional array
  Selector2 : Selector  IndexOptions=Starting and ending indices (port)  Indices=[1 3]  OutputSizes=1
  Selector3 : Selector  IndexOptions=Starting and ending indices (port)  Indices=[1 3]  OutputSizes=1
  k:m : Outport
  k:n : Outport  Port=2
  wires:
  Input/1 -> Matrix Concatenate3/1, Matrix Concatenate/1
  Selector3/1 -> k:m/1  "k:m"
  Selector2/1 -> k:n/1  "k:n"
  Constant6/1 -> Matrix Concatenate/2
  Matrix Concatenate/1 -> Selector3/2
  Constant7/1 -> Matrix Concatenate3/2
  Constant4/1 -> Selector2/1
  Matrix Concatenate3/1 -> Selector2/2
  Constant5/1 -> Selector3/1

== system HouseHolderTransformTest/Subsystem/Subsystem3/Subsystem1 ==
  In1 : Inport
  Abs : Abs  SaturateOnIntegerOverflow=off
  Abs1 : Abs  SaturateOnIntegerOverflow=off
  Complex to Real-Imag : ComplexToRealImag
  Constant : Constant  Value=0
  Constant1 : Constant  Value=0
  Real-Imag to Complex : RealImagToComplex
  Switch : Switch  Criteria=u2 > Threshold  Threshold=1e-10  SaturateOnIntegerOverflow=off  InputSameDT=off
  Switch1 : Switch  Criteria=u2 > Threshold  Threshold=1e-10  SaturateOnIntegerOverflow=off  InputSameDT=off
  output : Outport
  wires:
  In1/1 -> Complex to Real-Imag/1
  Complex to Real-Imag/1 -> Abs/1, Switch/1
  Constant/1 -> Switch/3
  Constant1/1 -> Switch1/3
  Complex to Real-Imag/2 -> Abs1/1, Switch1/1
  Switch/1 -> Real-Imag to Complex/1
  Switch1/1 -> Real-Imag to Complex/2
  Real-Imag to Complex/1 -> output/1
  Abs/1 -> Switch/2
  Abs1/1 -> Switch1/2

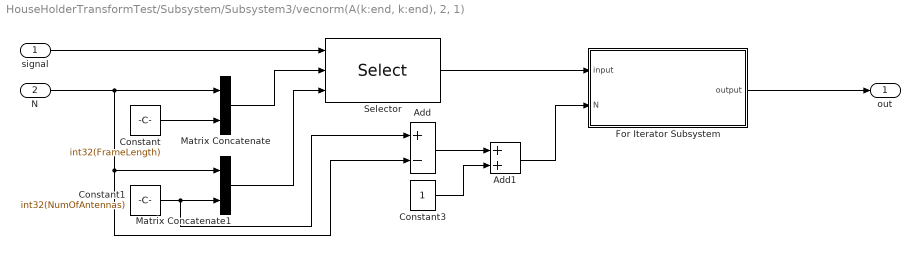
== system HouseHolderTransformTest/Subsystem/Subsystem3/vecnorm(A(k:end, k:end), 2, 1) ==
  signal : Inport
  N : Inport  Port=2
  Add : Sum  Inputs=+-
  Add1 : Sum
  Constant : Constant  Value=int32(FrameLength)  SampleTime=-1
  Constant1 : Constant  Value=int32(NumOfAntennas)  SampleTime=-1
  Constant3 : Constant
  For Iterator Subsystem : Subsystem  TreatAsAtomicUnit=on
  Matrix Concatenate : Concatenate
  Matrix Concatenate1 : Concatenate
  Selector : Selector  NumberOfDimensions=2  InputPortWidth=3  IndexOptions=Starting and ending indices (port),Starting and ending indices (port)  Indices=[1 3],1  OutputSizes=1,1
  out : Outport
  wires:
  Selector/1 -> For Iterator Subsystem/1(input)
  Add1/1 -> For Iterator Subsystem/2(N)
  For Iterator Subsystem/1(output) -> out/1
  Constant3/1 -> Add1/2
  Add/1 -> Add1/1
  N/1 -> Matrix Concatenate/1, Add/2, Matrix Concatenate1/1
  Constant1/1 -> Matrix Concatenate1/2, Add/1
  Matrix Concatenate1/1 -> Selector/3
  Constant/1 -> Matrix Concatenate/2
  Matrix Concatenate/1 -> Selector/2
  signal/1 -> Selector/1

== system HouseHolderTransformTest/Subsystem/Subsystem4/BLOCK A ==
  signal : Inport
  k : Inport  Port=2
  idx : Inport  Port=3
  MATLAB Function : MATLAB Function  TreatAsAtomicUnit=on
  A : Outport
  wires:
  signal/1 -> MATLAB Function/1("A ")
  MATLAB Function/1(A) -> A/1
  k/1 -> MATLAB Function/3(k)
  idx/1 -> MATLAB Function/2(idx)

== system HouseHolderTransformTest/Subsystem/Subsystem4/BLOCK B ==
  input : Inport
  2nd Norm : Subsystem
  If Action Subsystem : Subsystem  TreatAsAtomicUnit=on
  If Action Subsystem1 : Subsystem  TreatAsAtomicUnit=on
  Switch : Switch  Criteria=u2 ~= 0  AllowDiffInputSizes=on  SaturateOnIntegerOverflow=off  InputSameDT=off
  output : Outport
  wires:
  2nd Norm/1(output) -> If Action Subsystem/1(norm), Switch/2  "normX"
  If Action Subsystem/1(u) -> Switch/1
  Switch/1 -> output/1
  If Action Subsystem1/1(u) -> Switch/3
  input/1 -> 2nd Norm/1(input), If Action Subsystem/2(x), If Action Subsystem1/1(x)

== system HouseHolderTransformTest/Subsystem/Subsystem4/Subsystem ==
  Input : Inport
  Constant4 : Constant  Value=1:NumOfAntennas  OutDataTypeStr=int32  SampleTime=-1
  Constant5 : Constant  Value=1:FrameLength  OutDataTypeStr=int32  SampleTime=-1
  Constant6 : Constant  Value=FrameLength  OutDataTypeStr=int32
  Constant7 : Constant  Value=NumOfAntennas  OutDataTypeStr=int32
  Matrix Concatenate : Concatenate  Mode=Multidimensional array
  Matrix Concatenate3 : Concatenate  Mode=Multidimensional array
  Selector2 : Selector  IndexOptions=Starting and ending indices (port)  Indices=[1 3]  OutputSizes=1
  Selector3 : Selector  IndexOptions=Starting and ending indices (port)  Indices=[1 3]  OutputSizes=1
  k:m : Outport
  k:n : Outport  Port=2
  wires:
  Constant5/1 -> Selector3/1
  Matrix Concatenate3/1 -> Selector2/2
  Constant4/1 -> Selector2/1
  Constant7/1 -> Matrix Concatenate3/2
  Matrix Concatenate/1 -> Selector3/2
  Constant6/1 -> Matrix Concatenate/2
  Selector2/1 -> k:n/1  "k:n"
  Selector3/1 -> k:m/1  "k:m"
  Input/1 -> Matrix Concatenate/1, Matrix Concatenate3/1

== system HouseHolderTransformTest/Subsystem/Subsystem4/Subsystem1 ==
  In1 : Inport
  Abs : Abs  SaturateOnIntegerOverflow=off
  Abs1 : Abs  SaturateOnIntegerOverflow=off
  Complex to Real-Imag : ComplexToRealImag
  Constant : Constant  Value=0
  Constant1 : Constant  Value=0
  Real-Imag to Complex : RealImagToComplex
  Switch : Switch  Criteria=u2 > Threshold  Threshold=1e-10  SaturateOnIntegerOverflow=off  InputSameDT=off
  Switch1 : Switch  Criteria=u2 > Threshold  Threshold=1e-10  SaturateOnIntegerOverflow=off  InputSameDT=off
  output : Outport
  wires:
  Abs1/1 -> Switch1/2
  Abs/1 -> Switch/2
  Real-Imag to Complex/1 -> output/1
  Switch1/1 -> Real-Imag to Complex/2
  Switch/1 -> Real-Imag to Complex/1
  Complex to Real-Imag/2 -> Switch1/1, Abs1/1
  Constant1/1 -> Switch1/3
  Constant/1 -> Switch/3
  Complex to Real-Imag/1 -> Switch/1, Abs/1
  In1/1 -> Complex to Real-Imag/1

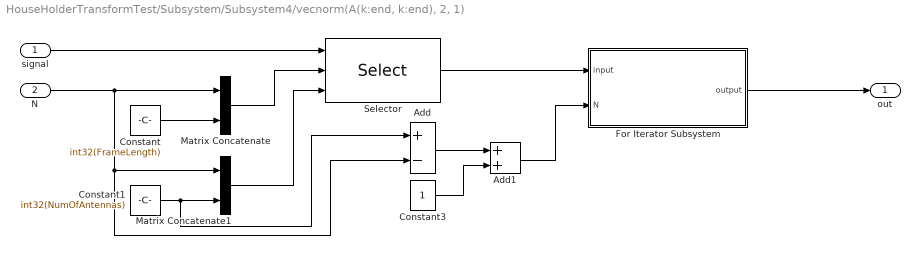
== system HouseHolderTransformTest/Subsystem/Subsystem4/vecnorm(A(k:end, k:end), 2, 1) ==
  signal : Inport
  N : Inport  Port=2
  Add : Sum  Inputs=+-
  Add1 : Sum
  Constant : Constant  Value=int32(FrameLength)  SampleTime=-1
  Constant1 : Constant  Value=int32(NumOfAntennas)  SampleTime=-1
  Constant3 : Constant
  For Iterator Subsystem : Subsystem  TreatAsAtomicUnit=on
  Matrix Concatenate : Concatenate
  Matrix Concatenate1 : Concatenate
  Selector : Selector  NumberOfDimensions=2  InputPortWidth=3  IndexOptions=Starting and ending indices (port),Starting and ending indices (port)  Indices=[1 3],1  OutputSizes=1,1
  out : Outport
  wires:
  signal/1 -> Selector/1
  Matrix Concatenate/1 -> Selector/2
  Constant/1 -> Matrix Concatenate/2
  Matrix Concatenate1/1 -> Selector/3
  Constant1/1 -> Add/1, Matrix Concatenate1/2
  N/1 -> Matrix Concatenate1/1, Add/2, Matrix Concatenate/1
  Add/1 -> Add1/1
  Constant3/1 -> Add1/2
  For Iterator Subsystem/1(output) -> out/1
  Add1/1 -> For Iterator Subsystem/2(N)
  Selector/1 -> For Iterator Subsystem/1(input)

== system HouseHolderTransformTest/For Iterator Subsystem1/Subsystem3/BLOCK B/2nd Norm ==
  input : Inport
  Add : Sum
  Complex to Real-Imag : ComplexToRealImag
  Sqrt : Sqrt
  Square : Math  Operator=square  SignedPower=on  RndMeth=Zero
  Square1 : Math  Operator=square  SignedPower=on  RndMeth=Zero
  Sum of Elements : Sum  Inputs=+
  output : Outport
  wires:
  Square1/1 -> Add/2
  Sum of Elements/1 -> Sqrt/1
  Add/1 -> Sum of Elements/1
  Square/1 -> Add/1
  Complex to Real-Imag/1 -> Square/1
  Sqrt/1 -> output/1
  Complex to Real-Imag/2 -> Square1/1
  input/1 -> Complex to Real-Imag/1

== system HouseHolderTransformTest/For Iterator Subsystem1/Subsystem3/BLOCK B/If Action Subsystem ==
  norm : Inport
  x : Inport  Port=2
  Assignment : Assignment  IndexOptions=Index vector (dialog)  Indices=1  OutputSizes=1
  Divide : Subsystem  Tag=DecoupledSystem
  Divide1 : Subsystem  Tag=DecoupledSystem
  Selector : Selector  NumberOfDimensions=2  InputPortWidth=FrameLength  IndexOptions=Starting index (dialog),Index vector (dialog)  Indices=1,1  OutputSizes=1,1
  Sqrt : Sqrt
  Subsystem Reference : Subsystem  ReferencedSubsystem=CompAbs
  getU(1) : Subsystem
  u : Outport
  wires:
  Sqrt/1 -> Divide1/2(In2)
  Selector/1 -> getU(1)/1(input)  "u1"
  x/1 -> Divide/1(In1)
  norm/1 -> Divide/2(In2)
  Divide/1(Out1) -> Selector/1, Assignment/1
  Divide1/1(Out1) -> u/1
  Subsystem Reference/1 -> Sqrt/1
  Assignment/1 -> Divide1/1(In1)
  getU(1)/1(u(1)) -> Assignment/2, Subsystem Reference/1  "u1"

== system HouseHolderTransformTest/For Iterator Subsystem1/Subsystem3/BLOCK B/If Action Subsystem1 ==
  x : Inport
  Assignment : Assignment  IndexOptions=Index vector (dialog)  Indices=1  OutputSizes=1
  Constant : Constant  Value=sqrt(2)
  u : Outport
  wires:
  x/1 -> Assignment/1
  Constant/1 -> Assignment/2
  Assignment/1 -> u/1

== system HouseHolderTransformTest/For Iterator Subsystem1/Subsystem3/vecnorm(A(k:end, k:end), 2, 1)/For Iterator Subsystem ==
  input : Inport
  N : Inport  Port=2
  2nd Norm : Subsystem
  Assignment : Assignment  IndexOptions=Index vector (port)  Indices=1  OutputSizes=1
  Constant : Constant  Value=zeros(1 , NumOfAntennas)
  For Iterator : ForIterator  IterationSource=external
  Selector : Selector  NumberOfDimensions=2  InputPortWidth=3  IndexOptions=Select all,Index vector (port)  Indices=[1 3],1  OutputSizes=1,1
  output : Outport
  wires:
  Assignment/1 -> output/1
  2nd Norm/1(output) -> Assignment/2
  Constant/1 -> Assignment/1
  N/1 -> For Iterator/1
  Selector/1 -> 2nd Norm/1(input)
  For Iterator/1 -> Selector/2, Assignment/3
  input/1 -> Selector/1

== system HouseHolderTransformTest/Subsystem/Subsystem1/BLOCK B/2nd Norm ==
  input : Inport
  Add : Sum
  Complex to Real-Imag : ComplexToRealImag
  Sqrt : Sqrt
  Square : Math  Operator=square  SignedPower=on  RndMeth=Zero
  Square1 : Math  Operator=square  SignedPower=on  RndMeth=Zero
  Sum of Elements : Sum  Inputs=+
  output : Outport
  wires:
  input/1 -> Complex to Real-Imag/1
  Complex to Real-Imag/2 -> Square1/1
  Sqrt/1 -> output/1
  Complex to Real-Imag/1 -> Square/1
  Square/1 -> Add/1
  Add/1 -> Sum of Elements/1
  Sum of Elements/1 -> Sqrt/1
  Square1/1 -> Add/2

== system HouseHolderTransformTest/Subsystem/Subsystem1/BLOCK B/If Action Subsystem ==
  norm : Inport
  x : Inport  Port=2
  Assignment : Assignment  IndexOptions=Index vector (dialog)  Indices=1  OutputSizes=1
  Divide : Subsystem  Tag=DecoupledSystem
  Divide1 : Subsystem  Tag=DecoupledSystem
  Selector : Selector  NumberOfDimensions=2  InputPortWidth=FrameLength  IndexOptions=Starting index (dialog),Index vector (dialog)  Indices=1,1  OutputSizes=1,1
  Sqrt : Sqrt
  Subsystem Reference : Subsystem  ReferencedSubsystem=CompAbs
  getU(1) : Subsystem
  u : Outport
  wires:
  getU(1)/1(u(1)) -> Subsystem Reference/1, Assignment/2  "u1"
  Assignment/1 -> Divide1/1(In1)
  Subsystem Reference/1 -> Sqrt/1
  Divide1/1(Out1) -> u/1
  Divide/1(Out1) -> Assignment/1, Selector/1
  norm/1 -> Divide/2(In2)
  x/1 -> Divide/1(In1)
  Selector/1 -> getU(1)/1(input)  "u1"
  Sqrt/1 -> Divide1/2(In2)

== system HouseHolderTransformTest/Subsystem/Subsystem1/BLOCK B/If Action Subsystem1 ==
  x : Inport
  Assignment : Assignment  IndexOptions=Index vector (dialog)  Indices=1  OutputSizes=1
  Constant : Constant  Value=sqrt(2)
  u : Outport
  wires:
  Assignment/1 -> u/1
  Constant/1 -> Assignment/2
  x/1 -> Assignment/1

== system HouseHolderTransformTest/Subsystem/Subsystem1/vecnorm(A(k:end, k:end), 2, 1)/For Iterator Subsystem ==
  input : Inport
  N : Inport  Port=2
  2nd Norm : Subsystem
  Assignment : Assignment  IndexOptions=Index vector (port)  Indices=1  OutputSizes=1
  Constant : Constant  Value=zeros(1 , NumOfAntennas)
  For Iterator : ForIterator  IterationSource=external
  Selector : Selector  NumberOfDimensions=2  InputPortWidth=3  IndexOptions=Select all,Index vector (port)  Indices=[1 3],1  OutputSizes=1,1
  output : Outport
  wires:
  input/1 -> Selector/1
  For Iterator/1 -> Assignment/3, Selector/2
  Selector/1 -> 2nd Norm/1(input)
  N/1 -> For Iterator/1
  Constant/1 -> Assignment/1
  2nd Norm/1(output) -> Assignment/2
  Assignment/1 -> output/1

== system HouseHolderTransformTest/Subsystem/Subsystem2/BLOCK B/2nd Norm ==
  input : Inport
  Add : Sum
  Complex to Real-Imag : ComplexToRealImag
  Sqrt : Sqrt
  Square : Math  Operator=square  SignedPower=on  RndMeth=Zero
  Square1 : Math  Operator=square  SignedPower=on  RndMeth=Zero
  Sum of Elements : Sum  Inputs=+
  output : Outport
  wires:
  Square1/1 -> Add/2
  Sum of Elements/1 -> Sqrt/1
  Add/1 -> Sum of Elements/1
  Square/1 -> Add/1
  Complex to Real-Imag/1 -> Square/1
  Sqrt/1 -> output/1
  Complex to Real-Imag/2 -> Square1/1
  input/1 -> Complex to Real-Imag/1

== system HouseHolderTransformTest/Subsystem/Subsystem2/BLOCK B/If Action Subsystem ==
  norm : Inport
  x : Inport  Port=2
  Assignment : Assignment  IndexOptions=Index vector (dialog)  Indices=1  OutputSizes=1
  Divide : Subsystem  Tag=DecoupledSystem
  Divide1 : Subsystem  Tag=DecoupledSystem
  Selector : Selector  NumberOfDimensions=2  InputPortWidth=FrameLength  IndexOptions=Starting index (dialog),Index vector (dialog)  Indices=1,1  OutputSizes=1,1
  Sqrt : Sqrt
  Subsystem Reference : Subsystem  ReferencedSubsystem=CompAbs
  getU(1) : Subsystem
  u : Outport
  wires:
  Sqrt/1 -> Divide1/2(In2)
  Selector/1 -> getU(1)/1(input)  "u1"
  x/1 -> Divide/1(In1)
  norm/1 -> Divide/2(In2)
  Divide/1(Out1) -> Selector/1, Assignment/1
  Divide1/1(Out1) -> u/1
  Subsystem Reference/1 -> Sqrt/1
  Assignment/1 -> Divide1/1(In1)
  getU(1)/1(u(1)) -> Assignment/2, Subsystem Reference/1  "u1"

== system HouseHolderTransformTest/Subsystem/Subsystem2/BLOCK B/If Action Subsystem1 ==
  x : Inport
  Assignment : Assignment  IndexOptions=Index vector (dialog)  Indices=1  OutputSizes=1
  Constant : Constant  Value=sqrt(2)
  u : Outport
  wires:
  x/1 -> Assignment/1
  Constant/1 -> Assignment/2
  Assignment/1 -> u/1

== system HouseHolderTransformTest/Subsystem/Subsystem2/vecnorm(A(k:end, k:end), 2, 1)/For Iterator Subsystem ==
  input : Inport
  N : Inport  Port=2
  2nd Norm : Subsystem
  Assignment : Assignment  IndexOptions=Index vector (port)  Indices=1  OutputSizes=1
  Constant : Constant  Value=zeros(1 , NumOfAntennas)
  For Iterator : ForIterator  IterationSource=external
  Selector : Selector  NumberOfDimensions=2  InputPortWidth=3  IndexOptions=Select all,Index vector (port)  Indices=[1 3],1  OutputSizes=1,1
  output : Outport
  wires:
  Assignment/1 -> output/1
  2nd Norm/1(output) -> Assignment/2
  Constant/1 -> Assignment/1
  N/1 -> For Iterator/1
  Selector/1 -> 2nd Norm/1(input)
  For Iterator/1 -> Selector/2, Assignment/3
  input/1 -> Selector/1

== system HouseHolderTransformTest/Subsystem/Subsystem3/BLOCK B/2nd Norm ==
  input : Inport
  Add : Sum
  Complex to Real-Imag : ComplexToRealImag
  Sqrt : Sqrt
  Square : Math  Operator=square  SignedPower=on  RndMeth=Zero
  Square1 : Math  Operator=square  SignedPower=on  RndMeth=Zero
  Sum of Elements : Sum  Inputs=+
  output : Outport
  wires:
  Square1/1 -> Add/2
  Sum of Elements/1 -> Sqrt/1
  Add/1 -> Sum of Elements/1
  Square/1 -> Add/1
  Complex to Real-Imag/1 -> Square/1
  Sqrt/1 -> output/1
  Complex to Real-Imag/2 -> Square1/1
  input/1 -> Complex to Real-Imag/1

== system HouseHolderTransformTest/Subsystem/Subsystem3/BLOCK B/If Action Subsystem ==
  norm : Inport
  x : Inport  Port=2
  Assignment : Assignment  IndexOptions=Index vector (dialog)  Indices=1  OutputSizes=1
  Divide : Subsystem  Tag=DecoupledSystem
  Divide1 : Subsystem  Tag=DecoupledSystem
  Selector : Selector  NumberOfDimensions=2  InputPortWidth=FrameLength  IndexOptions=Starting index (dialog),Index vector (dialog)  Indices=1,1  OutputSizes=1,1
  Sqrt : Sqrt
  Subsystem Reference : Subsystem  ReferencedSubsystem=CompAbs
  getU(1) : Subsystem
  u : Outport
  wires:
  Sqrt/1 -> Divide1/2(In2)
  Selector/1 -> getU(1)/1(input)  "u1"
  x/1 -> Divide/1(In1)
  norm/1 -> Divide/2(In2)
  Divide/1(Out1) -> Selector/1, Assignment/1
  Divide1/1(Out1) -> u/1
  Subsystem Reference/1 -> Sqrt/1
  Assignment/1 -> Divide1/1(In1)
  getU(1)/1(u(1)) -> Assignment/2, Subsystem Reference/1  "u1"

== system HouseHolderTransformTest/Subsystem/Subsystem3/BLOCK B/If Action Subsystem1 ==
  x : Inport
  Assignment : Assignment  IndexOptions=Index vector (dialog)  Indices=1  OutputSizes=1
  Constant : Constant  Value=sqrt(2)
  u : Outport
  wires:
  x/1 -> Assignment/1
  Constant/1 -> Assignment/2
  Assignment/1 -> u/1
